simulink model "sgMdl_Serial_Onboard_RS232Loopback"  (R2024b)
settings: Solver=FixedStepAuto  StartTime=0.0  StopTime=inf  RelTol=1e-3  EnableMultiTasking=on
libraries: slrealtimeseriallib x6, speedgoatlib_serial_onboard x5, simulink x3, slrealtimeutilitieslib x2
Description:
  | Serial - Onboard RS-232 Loopback
settings Model: ModifiedByFormat=Speedgoat  SimulationMode=external  ExtModeTrigDuration=100000  Creator=Speedgoat  LastModifiedBy=Speedgoat
settings SolverCC: ConcurrentTasks=on  AlgebraicLoopSolver=TrustRegion  PositivePriorityOrder=on  InsertRTBMode=Never (minimum delay)
settings DataIOCC: LimitDataPoints=on  SaveFormat=Array  SignalLoggingSaveFormat=ModelDataLogs  ReturnWorkspaceOutputs=off
settings OptimizationCC: BlockReduction=off  OptimizeBlockIOStorage=off  BufferReuse=off  GlobalBufferReuse=off  ExpressionFolding=off  ExpressionDepthLimit=2147483647  LocalBlockOutputs=off  OptimizeDataStoreBuffers=off  BusAssignmentInplaceUpdate=off
settings DebuggingCC: UnderspecifiedInitializationDetection=Classic  MergeDetectMultiDrivingBlocksExec=none  SolverPrmCheckMsg=warning  TasksWithSamePriorityMsg=none  FcnCallInpInsideContextMsg=warning  StateNameClashWarn=warning  SFUnexpectedBacktrackingDiag=warning  SFNoUnconditionalDefaultTransitionDiag=warning  SFExecutionAtInitializationDiag=none  ArithmeticOperatorsInVariantConditions=warning
settings HardwareCC: ProdBitPerLong=64  ProdLongLongMode=on  ProdHWDeviceType=Intel->x86-64 (Linux 64)
settings ModelReferenceCC: EnableRefExpFcnMdlSchedulingChecks=on  PropagateSignalLabelsOutOfModel=off
settings SFSimCC: SimUseLocalCustomCode=off  CustomCodeUndefinedFunction=UseInterfaceOnly
settings RTWCC: Description=Speedgoat Real-Time Target Machine  SystemTargetFile=speedgoat.tlc  TemplateMakefile=slrealtime_default_tmf  RTWUseLocalCustomCode=off  Toolchain=Simulink Real-Time Toolchain  BuildConfiguration=Faster Runs  TargetLang=C++  GPUComputeCapability=3.5  DLArmComputeVersion=19.05
settings CodeAppCC: StateflowObjectComments=on
settings SimulinkRealTimeTargetCC: SubcomponentCodeInterfacePackaging=Reusable function  InstructionSetFMA=off  LogToMDFFile=off  SLRTFileLogMaxRuns=10
settings ConfigComp: CovMetricSettings=dw  CovSaveCumulativeToWorkspaceVar=on  CovSaveSingleToWorkspaceVar=on  CovExternalEMLEnable=off  CovSFcnEnable=off  CovBoundaryAbsTol=1.0e-5

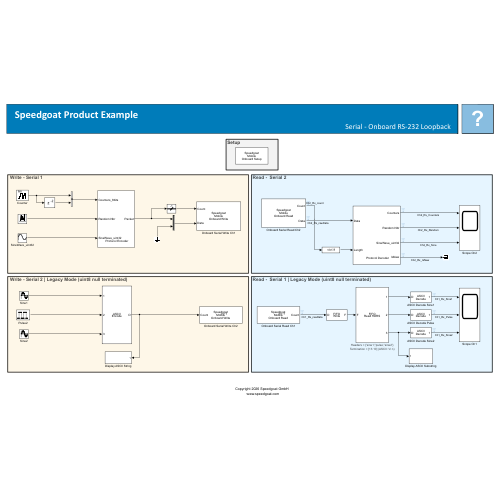
[thumbnail: Simulink's stored preview of the top-level diagram]
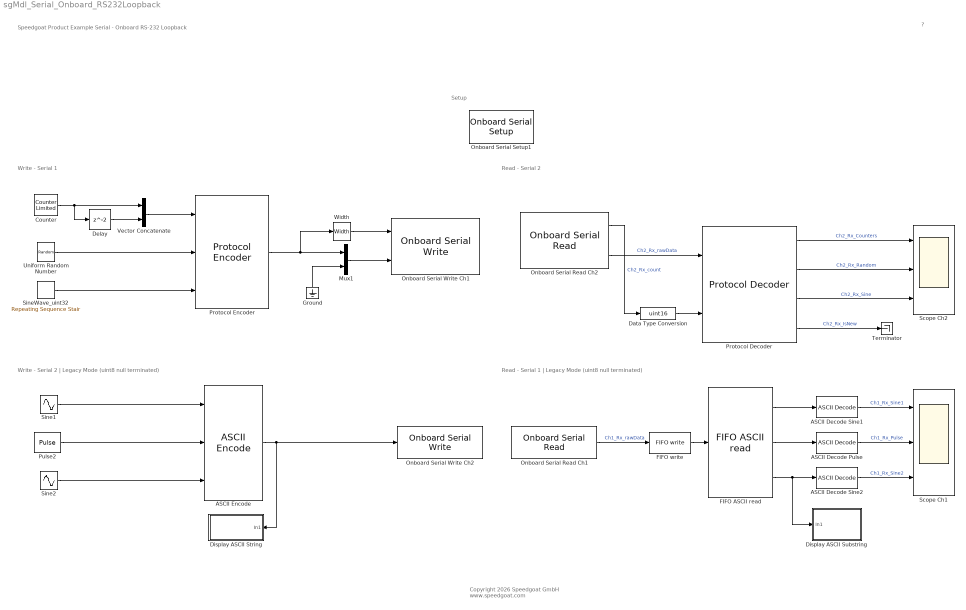
== system sgMdl_Serial_Onboard_RS232Loopback ==
  note: Setup
  note: Read - Serial 2
  note: Write - Serial 1
  note: Write - Serial 2 | Legacy Mode (uint8 null terminated)
  note: Read - Serial 1 | Legacy Mode (uint8 null terminated)
  note: Speedgoat Product Example
      | Serial - Onboard RS-232 Loopback
  note: ?
  note: Copyright 2026 Speedgoat GmbH
      |  www.speedgoat.com
  ASCII Decode Pulse : slrealtimeseriallib/ASCII Decode  format=pulse %d\r\n  nvars=1  vartypes={ }
  ASCII Decode Sine1 : slrealtimeseriallib/ASCII Decode  format=sine1 %f\r\n  nvars=1  vartypes={'double'}
  ASCII Decode Sine2 : slrealtimeseriallib/ASCII Decode  format=sine2 %f\r\n  nvars=1  vartypes={ }
  ASCII Encode : slrealtimeseriallib/ASCII Encode  format=START foo sine1 %f\r\n bar pulse %d\r\n fud sine2 %f\r\n  nvars=3  maxlength=128  vartypes={ 'double' }
  Counter : simulink/Sources/Counter Limited  uplimit=100  tsamp=-1
  Data Type Conversion : DataTypeConversion  OutDataTypeStr=uint16  SaturateOnIntegerOverflow=off  RndMeth=Floor
  Delay : Delay
  Display ASCII String : Subsystem
  Display ASCII Substring : Subsystem
  FIFO ASCII read : slrealtimeseriallib/FIFO ASCII read  header={'sine1','pulse','sine2'}  term=[13 10]  hold=Hold last output if no new data  enable=off  maxsize=128  outputtype=8 bit uint null terminated  sampletime=-1
      settings: AttributesFormatString=|
      | Headers = %<header>
      | Termination = %<term> (ASCII: \r\ n)
  FIFO write : slrealtimeseriallib/FIFO write  size=255  inputtype=8 bit uint null terminated  present=off  sampletime=-1  id=FIFO overflow: Block for Ch1 Rx
  Ground : Ground
  Mux1 : Mux  Inputs=2
  Onboard Serial Read Ch1 : speedgoatlib_serial_onboard/Onboard Serial Read  parMachineType=Performance  parPort=1  parSampleTime=0.01  parEnLegacy=on  parDataType=8 bit uint null terminated  parRxSwFifoSize=128
      settings: SourceProductName=Onboard
  Onboard Serial Read Ch2 : speedgoatlib_serial_onboard/Onboard Serial Read  parMachineType=Performance  parPort=2  parSampleTime=0.01  parEnLegacy=off  parDataType=count+16 bit int  parRxSwFifoSize=128
      settings: SourceProductName=Onboard
  Onboard Serial Setup1 : speedgoatlib_serial_onboard/Onboard Serial Setup  parMachineType=Performance  parPort1=RS232  parPort2=RS232  parPort3=Disabled  parPort4=Disabled  parEnCustBaud1=off  parCustBaudValue1=9600  parBaud1=115200  parParity1=None  parDataBits1=8  parStopBits1=1  parTxSwFifoSize1=128  parRxSwFifoSize1=128  parCtsMode1=off  parTerm1=on  parEnCustBaud2=off  parCustBaudValue2=9600  parBaud2=115200  parParity2=None  parDataBits2=8  parStopBits2=1  parTxSwFifoSize2=128  parRxSwFifoSize2=128  parCtsMode2=off  parTerm2=on  parEnCustBaud3=on  parCustBaudValue3=9600  parBaud3=115200  parParity3=None  parDataBits3=8  parStopBits3=1  parTxSwFifoSize3=64  parRxSwFifoSize3=64  parCtsMode3=on  parTerm3=on  parEnCustBaud4=on  parCustBaudValue4=9600  parBaud4=115200  parParity4=None  parDataBits4=8  parStopBits4=1  parTxSwFifoSize4=64  parRxSwFifoSize4=64  parCtsMode4=on  parTerm4=on
      settings: SourceProductName=Onboard
  Onboard Serial Write Ch1 : speedgoatlib_serial_onboard/Onboard Serial Write  parMachineType=Performance  parPort=1  parSampleTime=0.01  parEnLegacy=off  parDataType=count+16 bit int  parMdlStopMsgEnable=off  parMdlStopMsgData=['CONF' char(13)]  parMdlStopFifoOptions=Write to TX FIFO directly  parMdlStopMsgsDataArr=[67 79 78 70 13]  parMdlStopMsgsDataSize=5  parTxSwFifoSize=128
      settings: SourceProductName=Onboard
  Onboard Serial Write Ch2 : speedgoatlib_serial_onboard/Onboard Serial Write  parMachineType=Performance  parPort=2  parSampleTime=0.01  parEnLegacy=on  parDataType=8 bit uint null terminated  parMdlStopMsgEnable=off  parMdlStopMsgData=['CONF' char(13)]  parMdlStopFifoOptions=Write to TX FIFO directly  parMdlStopMsgsDataArr=[67 79 78 70 13]  parMdlStopMsgsDataSize=5  parTxSwFifoSize=128
      settings: SourceProductName=Onboard
  Protocol Decoder : slrealtimeutilitieslib/Protocol Decoder  IsParseCSV=off  Header='START'  FieldTable={ 'Counters', '2', 'uint8', 'Little endian'; 'Random Nbr', '1', 'double', 'Little endian'; 'SineWave_uint32', '1', 'uint32', 'Little endian' }  IsVariableSizeLastField=off  MaxVariableSizeFieldLength=[]  IsChecksumRequired=off  ChecksumAlgorithm=XOR of bytes  ChecksumSize=[]  TerminatorOption=<none>  CustomTerminatorVal=[]  IsInputLengthAvailable=on
  Protocol Encoder : slrealtimeutilitieslib/Protocol Encoder  Header='START'  FieldTable={ 'Counters_8bits', '2', 'uint8', 'Little endian'; 'Random Nbr', '1', 'double', 'Little endian'; 'SineWave_uint32', '1', 'uint32', 'Little endian' }  IsChecksumRequired=off  ChecksumAlgorithm=XOR of bytes  ChecksumSize=[]  TerminatorOption=<none>  CustomTerminatorVal=[]
  Pulse2 : DiscretePulseGenerator  Period=101  PulseWidth=50  SampleTime=0.01
  Scope Ch1 : Scope  NumInputPorts=3
  Scope Ch2 : Scope  NumInputPorts=3
  Sine1 : Sin  Amplitude=2  Bias=4  Frequency=10.1  SampleTime=0.01
  Sine2 : Sin  Bias=-2  Frequency=10.11  Phase=3.14  SampleTime=0.01
  SineWave_uint32 : simulink/Sources/Repeating Sequence Stair  OutValues=uint32((2^31-1) * sin(2*pi*(0:99)/100) + 2^31)  tsamp=-1  OutMin=[]  OutMax=[]  OutDataTypeStr=uint32  OutputDataTypeScalingMode=uint32  OutDataType=fixdt(0,8)  ConRadixGroup=Best Precision: Vector-wise  OutScaling=2^-12
  Terminator : Terminator
  Uniform Random Number : UniformRandomNumber  Minimum=0  Maximum=100  SampleTime=0.01
  Vector Concatenate : Concatenate
  Width : Width  DataType=uint32
  wires:
  Mux1/1 -> Onboard Serial Write Ch1/2
  Width/1 -> Onboard Serial Write Ch1/1
  Onboard Serial Read Ch2/2 -> Protocol Decoder/1  "Ch2_Rx_rawData"
  Ground/1 -> Mux1/2
  Pulse2/1 -> ASCII Encode/2
  Sine2/1 -> ASCII Encode/3
  Sine1/1 -> ASCII Encode/1
  ASCII Encode/1 -> Display ASCII String/1(In1), Onboard Serial Write Ch2/1
  Onboard Serial Read Ch1/1 -> FIFO write/1  "Ch1_Rx_rawData"
  FIFO ASCII read/1 -> ASCII Decode Sine1/1
  ASCII Decode Pulse/1 -> Scope Ch1/2  "Ch1_Rx_Pulse"
  FIFO ASCII read/3 -> Display ASCII Substring/1(In1), ASCII Decode Sine2/1
  ASCII Decode Sine1/1 -> Scope Ch1/1  "Ch1_Rx_Sine1"
  FIFO ASCII read/2 -> ASCII Decode Pulse/1
  FIFO write/1 -> FIFO ASCII read/1
  ASCII Decode Sine2/1 -> Scope Ch1/3  "Ch1_Rx_Sine2"
  Uniform Random Number/1 -> Protocol Encoder/2
  Counter/1 -> Delay/1, Vector Concatenate/1
  Protocol Encoder/1 -> Mux1/1, Width/1
  SineWave_uint32/1 -> Protocol Encoder/3
  Vector Concatenate/1 -> Protocol Encoder/1
  Delay/1 -> Vector Concatenate/2
  Protocol Decoder/4 -> Terminator/1  "Ch2_Rx_IsNew"
  Onboard Serial Read Ch2/1 -> Data Type Conversion/1  "Ch2_Rx_count"
  Protocol Decoder/1 -> Scope Ch2/1  "Ch2_Rx_Counters"
  Protocol Decoder/2 -> Scope Ch2/2  "Ch2_Rx_Random"
  Protocol Decoder/3 -> Scope Ch2/3  "Ch2_Rx_Sine"
  Data Type Conversion/1 -> Protocol Decoder/2

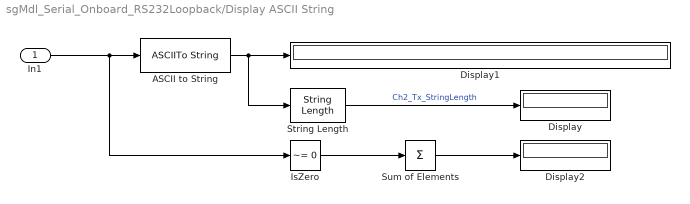
== system sgMdl_Serial_Onboard_RS232Loopback/Display ASCII String ==
  In1 : Inport
  ASCII to String : ASCIIToString
  Display : Display
  Display1 : Display
  Display2 : Display
  IsZero : simulink/Logic and Bit Operations/Compare To Zero  relop=~=  OutDataTypeStr=boolean
      settings: LibrarySourceBlock=|
      | simulink/Quick Insert/Logic and Bit
      | Operations/IsZero
  String Length : StringLength
  Sum of Elements : Sum  Inputs=+
  wires:
  ASCII to String/1 -> String Length/1, Display1/1
  String Length/1 -> Display/1  "Ch2_Tx_StringLength"
  In1/1 -> IsZero/1, ASCII to String/1
  Sum of Elements/1 -> Display2/1
  IsZero/1 -> Sum of Elements/1

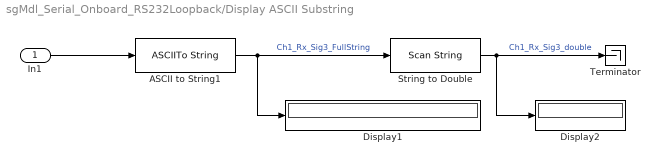
== system sgMdl_Serial_Onboard_RS232Loopback/Display ASCII Substring ==
  In1 : Inport
  ASCII to String1 : ASCIIToString
  Display1 : Display
  Display2 : Display
  String to Double : ScanString  Format="\"sine2 %lf\\r\\n\""
  Terminator : Terminator
  wires:
  In1/1 -> ASCII to String1/1
  ASCII to String1/1 -> String to Double/1, Display1/1  "Ch1_Rx_Sig3_FullString"
  String to Double/1 -> Terminator/1, Display2/1  "Ch1_Rx_Sig3_double"
